simulink model "tesst"  (R2017b)
settings: Solver=FixedStepAuto  StartTime=0.0  StopTime=20  FixedStep=0.01  RelTol=1e-3
settings Model: Creator=DELL  LastModifiedBy=DELL

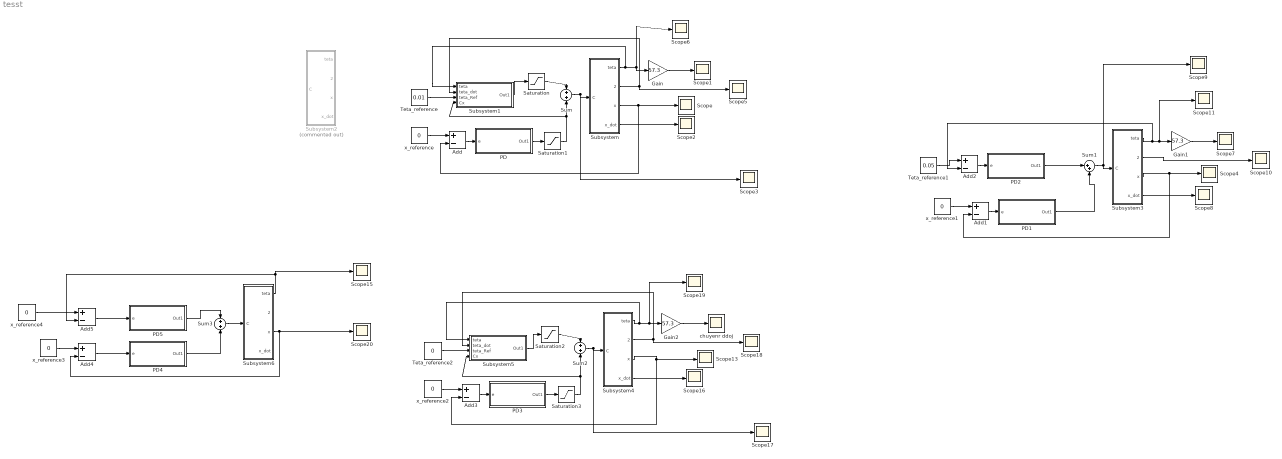
== system tesst ==
  Add{,1..5} (6 alike) : Sum  Inputs=+-
  Gain : Gain  Gain=57.3
  Gain1 : Gain  Gain=57.3
  Gain2 : Gain  Gain=57.3
  PD : Subsystem
  PD1 : Subsystem
  PD2 : Subsystem
  PD3 : Subsystem
  PD4 : Subsystem
  PD5 : Subsystem
  Saturation : Saturate  UpperLimit=0.8  LowerLimit=-0.8
  Saturation1 : Saturate  UpperLimit=0.2  LowerLimit=-0.2
  Saturation2 : Saturate  UpperLimit=0.7  LowerLimit=-0.7
  Saturation3 : Saturate  UpperLimit=0.25  LowerLimit=-0.25
  Scope{,1..11,13,15..20} (19 alike) : Scope
  Subsystem : Subsystem
  Subsystem1 : Subsystem
  Subsystem2 : Subsystem  Commented=on
  Subsystem3 : Subsystem
  Subsystem4 : Subsystem
  Subsystem5 : Subsystem
  Subsystem6 : Subsystem
  Sum : Sum
  Sum1 : Sum  Inputs=|++
  Sum2 : Sum
  Sum3 : Sum
  Teta_reference : Constant  Value=0.01
  Teta_reference1 : Constant  Value=0.05
  Teta_reference2 : Constant  Value=0
  chuyenr ddoj : Scope
  x_reference{,1..4} (5 alike) : Constant  Value=0
  wires:
  Subsystem/1(teta) -> Scope6/1, Gain/1, Subsystem1/1(teta)
  Subsystem/2(teta_dot) -> Subsystem1/2(teta_dot), Scope5/1
  Teta_reference/1 -> Subsystem1/3(teta_Ref)
  Subsystem/3(x) -> Add/2, Scope/1
  Subsystem/4(x_dot) -> Scope2/1
  Gain/1 -> Scope1/1
  x_reference/1 -> Add/1
  Add/1 -> PD/1(e)
  Sum/1 -> Scope3/1, Subsystem/1(C)
  Subsystem3/4(x_dot) -> Scope8/1
  Subsystem3/2(teta_dot) -> Scope10/1
  Gain1/1 -> Scope7/1
  Subsystem3/1(teta) -> Add2/2, Scope11/1, Gain1/1
  Subsystem3/3(x) -> Add1/2, Scope4/1
  Add1/1 -> PD1/1(e)
  Sum1/1 -> Scope9/1, Subsystem3/1(C)
  x_reference1/1 -> Add1/1
  PD1/1(Out1) -> Sum1/2
  PD2/1(Out1) -> Sum1/1
  Add2/1 -> PD2/1(e)
  Teta_reference1/1 -> Add2/1
  Subsystem1/1(Out1) -> Saturation/1
  Saturation/1 -> Sum/1
  PD/1(Out1) -> Saturation1/1
  Saturation1/1 -> Subsystem1/4(Cx), Sum/2
  Teta_reference2/1 -> Subsystem5/3(teta_Ref)
  Subsystem4/4(x_dot) -> Scope16/1
  Subsystem5/1(Out1) -> Saturation2/1
  Saturation2/1 -> Sum2/1
  Subsystem4/2(teta_dot) -> Subsystem5/2(teta_dot), Scope18/1
  Gain2/1 -> chuyenr ddoj/1
  Subsystem4/3(x) -> Add3/2, Scope13/1
  Subsystem4/1(teta) -> Scope19/1, Gain2/1, Subsystem5/1(teta)
  PD3/1(Out1) -> Saturation3/1
  Saturation3/1 -> Subsystem5/4(Cx), Sum2/2
  Add3/1 -> PD3/1(e)
  x_reference2/1 -> Add3/1
  Sum2/1 -> Scope17/1, Subsystem4/1(C)
  Add4/1 -> PD4/1(e)
  x_reference3/1 -> Add4/1
  Sum3/1 -> Subsystem6/1(C)
  PD4/1(Out1) -> Sum3/2
  Subsystem6/3(x) -> Scope20/1, Add4/2
  PD5/1(Out1) -> Sum3/1
  Add5/1 -> PD5/1(e)
  x_reference4/1 -> Add5/1
  Subsystem6/1(teta) -> Add5/2, Scope15/1

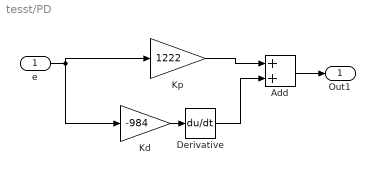
== system tesst/PD ==
  e : Inport
  Add : Sum
  Derivative : Derivative
  Kd : Gain  Gain=-984
  Kp : Gain  Gain=1222
  Out1 : Outport
  wires:
  Kp/1 -> Add/1
  e/1 -> Kd/1, Kp/1
  Add/1 -> Out1/1
  Kd/1 -> Derivative/1
  Derivative/1 -> Add/2

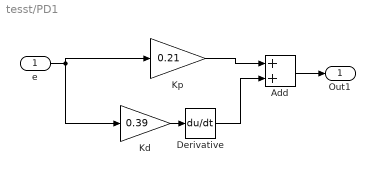
== system tesst/PD1 ==
  e : Inport
  Add : Sum
  Derivative : Derivative
  Kd : Gain  Gain=0.39
  Kp : Gain  Gain=0.21
  Out1 : Outport
  wires:
  Kp/1 -> Add/1
  e/1 -> Kd/1, Kp/1
  Add/1 -> Out1/1
  Kd/1 -> Derivative/1
  Derivative/1 -> Add/2

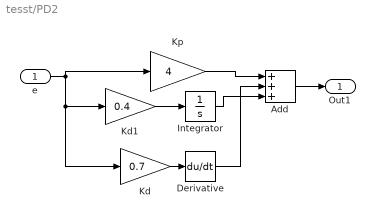
== system tesst/PD2 ==
  e : Inport
  Add : Sum  Inputs=+++
  Derivative : Derivative
  Integrator : Integrator
  Kd : Gain  Gain=0.7
  Kd1 : Gain  Gain=0.4
  Kp : Gain  Gain=4
  Out1 : Outport
  wires:
  Derivative/1 -> Add/2
  Kd/1 -> Derivative/1
  Add/1 -> Out1/1
  e/1 -> Kp/1, Kd1/1, Kd/1
  Kp/1 -> Add/1
  Kd1/1 -> Integrator/1
  Integrator/1 -> Add/3

== system tesst/PD3 ==
  e : Inport
  Add : Sum
  Derivative : Derivative
  Kd : Gain  Gain=0.39
  Kp : Gain  Gain=0.21
  Out1 : Outport
  wires:
  Kp/1 -> Add/1
  e/1 -> Kd/1, Kp/1
  Add/1 -> Out1/1
  Kd/1 -> Derivative/1
  Derivative/1 -> Add/2

== system tesst/PD4 ==
  e : Inport
  Add : Sum
  Derivative : Derivative
  Kd : Gain  Gain=0
  Kp : Gain  Gain=0
  Out1 : Outport
  wires:
  Kp/1 -> Add/1
  e/1 -> Kd/1, Kp/1
  Add/1 -> Out1/1
  Kd/1 -> Derivative/1
  Derivative/1 -> Add/2

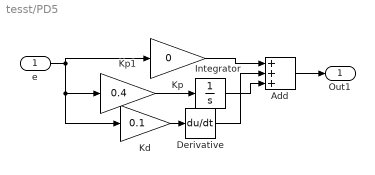
== system tesst/PD5 ==
  e : Inport
  Add : Sum  Inputs=+++
  Derivative : Derivative
  Integrator : Integrator
  Kd : Gain  Gain=0.1
  Kp : Gain  Gain=0
  Kp1 : Gain  Gain=0.4
  Out1 : Outport
  wires:
  Derivative/1 -> Add/2
  Kd/1 -> Derivative/1
  Add/1 -> Out1/1
  e/1 -> Kp/1, Kp1/1, Kd/1
  Kp/1 -> Add/1
  Kp1/1 -> Integrator/1
  Integrator/1 -> Add/3

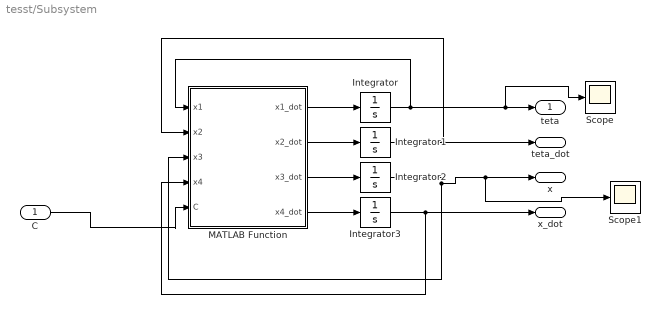
== system tesst/Subsystem ==
  C : Inport
  Integrator{,1..3} (4 alike) : Integrator
  MATLAB Function : MATLAB Function  TreatAsAtomicUnit=on
  Scope : Scope
  Scope1 : Scope
  teta : Outport
  teta_dot : Outport  Port=2
  x : Outport  Port=3
  x_dot : Outport  Port=4
  wires:
  MATLAB Function/2(x2_dot) -> Integrator1/1
  Integrator/1 -> teta/1, Scope/1, MATLAB Function/1(x1)
  MATLAB Function/4(x4_dot) -> Integrator3/1
  MATLAB Function/3(x3_dot) -> Integrator2/1
  MATLAB Function/1(x1_dot) -> Integrator/1
  Integrator1/1 -> teta_dot/1, MATLAB Function/2(x2)
  Integrator2/1 -> x/1, Scope1/1, MATLAB Function/3(x3)
  Integrator3/1 -> x_dot/1, MATLAB Function/4(x4)
  C/1 -> MATLAB Function/5(C)

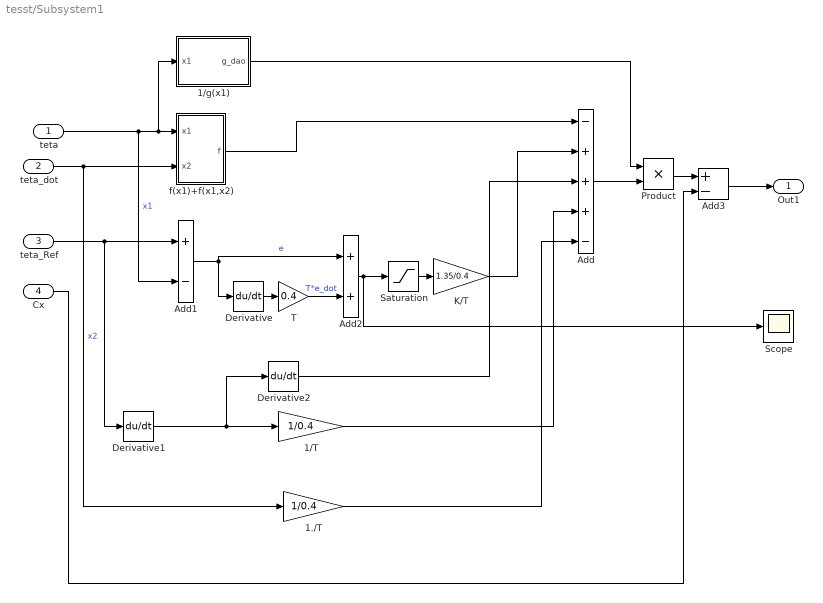
== system tesst/Subsystem1 ==
  teta : Inport
  teta_dot : Inport  Port=2
  teta_Ref : Inport  Port=3
  Cx : Inport  Port=4
  1./T : Gain  Gain=1/0.4
  1/T : Gain  Gain=1/0.4
  1/g(x1) : MATLAB Function  TreatAsAtomicUnit=on
  Add : Sum  Inputs=-+++-
  Add1 : Sum  Inputs=+-
  Add2 : Sum
  Add3 : Sum  Inputs=+-
  Derivative : Derivative
  Derivative1 : Derivative
  Derivative2 : Derivative
  K/T : Gain  Gain=1.35/0.4
  Product : Product
  Saturation : Saturate  UpperLimit=0.4  LowerLimit=-0.4
  Scope : Scope
  T : Gain  Gain=0.4
  f(x1)+f(x1,x2) : MATLAB Function  TreatAsAtomicUnit=on
  Out1 : Outport
  wires:
  teta_dot/1 -> 1./T/1, f(x1)+f(x1,x2)/2(x2)  "x2"
  teta/1 -> Add1/2, 1/g(x1)/1(x1), f(x1)+f(x1,x2)/1(x1)  "x1"
  1/g(x1)/1(g_dao) -> Product/1
  Add/1 -> Product/2
  f(x1)+f(x1,x2)/1(f) -> Add/1
  teta_Ref/1 -> Derivative1/1, Add1/1
  Derivative/1 -> T/1
  Add1/1 -> Derivative/1, Add2/1  "e"
  T/1 -> Add2/2  "T*e_dot"
  Add2/1 -> Scope/1, Saturation/1
  Saturation/1 -> K/T/1
  K/T/1 -> Add/2
  Derivative1/1 -> Derivative2/1, 1/T/1
  Derivative2/1 -> Add/3
  1/T/1 -> Add/4
  1./T/1 -> Add/5
  Product/1 -> Add3/1
  Cx/1 -> Add3/2
  Add3/1 -> Out1/1

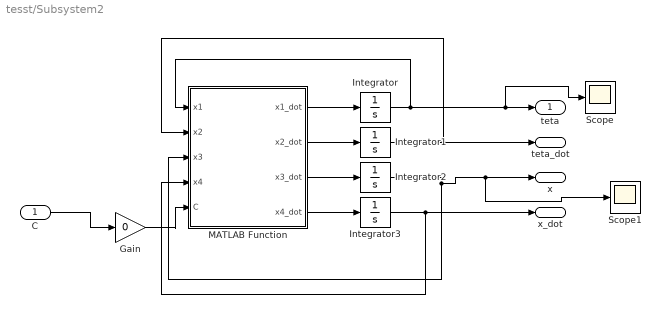
== system tesst/Subsystem2 ==
  C : Inport
  Gain : Gain  Gain=0
  Integrator : Integrator  InitialCondition=0.014
  Integrator1 : Integrator
  Integrator2 : Integrator  InitialCondition=0.03
  Integrator3 : Integrator
  MATLAB Function : MATLAB Function  TreatAsAtomicUnit=on
  Scope : Scope
  Scope1 : Scope
  teta : Outport
  teta_dot : Outport  Port=2
  x : Outport  Port=3
  x_dot : Outport  Port=4
  wires:
  MATLAB Function/2(x2_dot) -> Integrator1/1
  C/1 -> Gain/1
  Integrator/1 -> teta/1, Scope/1, MATLAB Function/1(x1)
  MATLAB Function/4(x4_dot) -> Integrator3/1
  MATLAB Function/3(x3_dot) -> Integrator2/1
  MATLAB Function/1(x1_dot) -> Integrator/1
  Integrator1/1 -> teta_dot/1, MATLAB Function/2(x2)
  Integrator2/1 -> x/1, Scope1/1, MATLAB Function/3(x3)
  Integrator3/1 -> x_dot/1, MATLAB Function/4(x4)
  Gain/1 -> MATLAB Function/5(C)

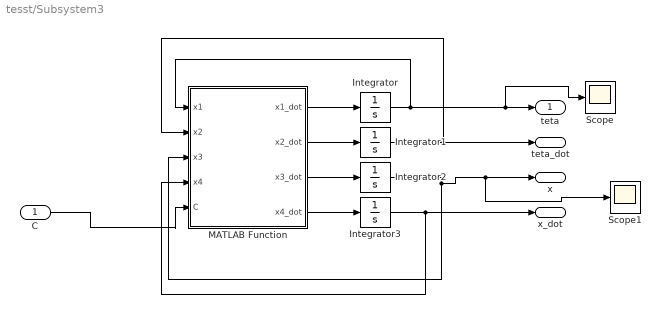
== system tesst/Subsystem3 ==
  C : Inport
  Integrator : Integrator  InitialCondition=0.014
  Integrator1 : Integrator
  Integrator2 : Integrator  InitialCondition=0.03
  Integrator3 : Integrator
  MATLAB Function : MATLAB Function  TreatAsAtomicUnit=on
  Scope : Scope
  Scope1 : Scope
  teta : Outport
  teta_dot : Outport  Port=2
  x : Outport  Port=3
  x_dot : Outport  Port=4
  wires:
  MATLAB Function/2(x2_dot) -> Integrator1/1
  Integrator/1 -> teta/1, Scope/1, MATLAB Function/1(x1)
  MATLAB Function/4(x4_dot) -> Integrator3/1
  MATLAB Function/3(x3_dot) -> Integrator2/1
  MATLAB Function/1(x1_dot) -> Integrator/1
  Integrator1/1 -> teta_dot/1, MATLAB Function/2(x2)
  Integrator2/1 -> x/1, Scope1/1, MATLAB Function/3(x3)
  Integrator3/1 -> x_dot/1, MATLAB Function/4(x4)
  C/1 -> MATLAB Function/5(C)

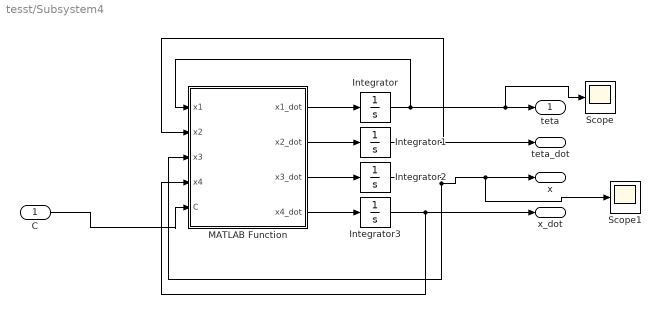
== system tesst/Subsystem4 ==
  C : Inport
  Integrator : Integrator  InitialCondition=0.017
  Integrator1 : Integrator
  Integrator2 : Integrator
  Integrator3 : Integrator
  MATLAB Function : MATLAB Function  TreatAsAtomicUnit=on
  Scope : Scope
  Scope1 : Scope
  teta : Outport
  teta_dot : Outport  Port=2
  x : Outport  Port=3
  x_dot : Outport  Port=4
  wires:
  MATLAB Function/2(x2_dot) -> Integrator1/1
  Integrator/1 -> teta/1, Scope/1, MATLAB Function/1(x1)
  MATLAB Function/4(x4_dot) -> Integrator3/1
  MATLAB Function/3(x3_dot) -> Integrator2/1
  MATLAB Function/1(x1_dot) -> Integrator/1
  Integrator1/1 -> teta_dot/1, MATLAB Function/2(x2)
  Integrator2/1 -> x/1, Scope1/1, MATLAB Function/3(x3)
  Integrator3/1 -> x_dot/1, MATLAB Function/4(x4)
  C/1 -> MATLAB Function/5(C)

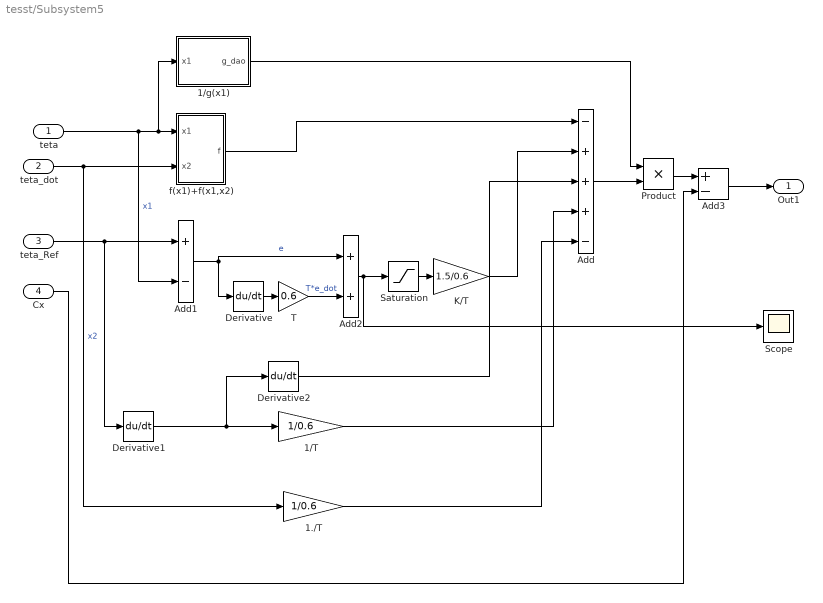
== system tesst/Subsystem5 ==
  teta : Inport
  teta_dot : Inport  Port=2
  teta_Ref : Inport  Port=3
  Cx : Inport  Port=4
  1./T : Gain  Gain=1/0.6
  1/T : Gain  Gain=1/0.6
  1/g(x1) : MATLAB Function  TreatAsAtomicUnit=on
  Add : Sum  Inputs=-+++-
  Add1 : Sum  Inputs=+-
  Add2 : Sum
  Add3 : Sum  Inputs=+-
  Derivative : Derivative
  Derivative1 : Derivative
  Derivative2 : Derivative
  K/T : Gain  Gain=1.5/0.6
  Product : Product
  Saturation : Saturate  UpperLimit=0.4  LowerLimit=-0.4
  Scope : Scope
  T : Gain  Gain=0.6
  f(x1)+f(x1,x2) : MATLAB Function  TreatAsAtomicUnit=on
  Out1 : Outport
  wires:
  teta_dot/1 -> 1./T/1, f(x1)+f(x1,x2)/2(x2)  "x2"
  teta/1 -> Add1/2, 1/g(x1)/1(x1), f(x1)+f(x1,x2)/1(x1)  "x1"
  1/g(x1)/1(g_dao) -> Product/1
  Add/1 -> Product/2
  f(x1)+f(x1,x2)/1(f) -> Add/1
  teta_Ref/1 -> Derivative1/1, Add1/1
  Derivative/1 -> T/1
  Add1/1 -> Derivative/1, Add2/1  "e"
  T/1 -> Add2/2  "T*e_dot"
  Add2/1 -> Scope/1, Saturation/1
  Saturation/1 -> K/T/1
  K/T/1 -> Add/2
  Derivative1/1 -> Derivative2/1, 1/T/1
  Derivative2/1 -> Add/3
  1/T/1 -> Add/4
  1./T/1 -> Add/5
  Product/1 -> Add3/1
  Cx/1 -> Add3/2
  Add3/1 -> Out1/1

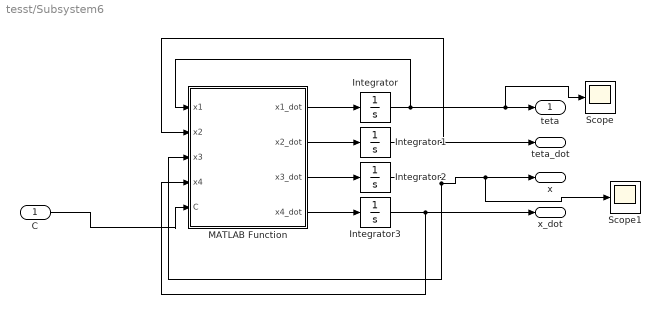
== system tesst/Subsystem6 ==
  C : Inport
  Integrator : Integrator  InitialCondition=0.017
  Integrator1 : Integrator
  Integrator2 : Integrator
  Integrator3 : Integrator
  MATLAB Function : MATLAB Function  TreatAsAtomicUnit=on
  Scope : Scope
  Scope1 : Scope
  teta : Outport
  teta_dot : Outport  Port=2
  x : Outport  Port=3
  x_dot : Outport  Port=4
  wires:
  MATLAB Function/2(x2_dot) -> Integrator1/1
  Integrator/1 -> teta/1, Scope/1, MATLAB Function/1(x1)
  MATLAB Function/4(x4_dot) -> Integrator3/1
  MATLAB Function/3(x3_dot) -> Integrator2/1
  MATLAB Function/1(x1_dot) -> Integrator/1
  Integrator1/1 -> teta_dot/1, MATLAB Function/2(x2)
  Integrator2/1 -> x/1, Scope1/1, MATLAB Function/3(x3)
  Integrator3/1 -> x_dot/1, MATLAB Function/4(x4)
  C/1 -> MATLAB Function/5(C)

== matlab function tesst/Subsystem1/f(x1)+f(x1,x2) ==
  data: x1 input; f output; x2 input
function f = fcn(x1,x2)
Mw=0.5;
Mb=7;
R=0.07;
L=0.3;
D=0.41;
g=9.8;
f=(-0.75*g*sin(x1)/L)/((0.75*(Mw*R+Mb*L*cos(x1))*cos(x1)/((2*Mw+Mb)*L))-1)+...
    (0.75*Mb*L*sin(x1)*cos(x1)*(x2^2)/(L*(2*Mw+Mb)))/((0.75*(Mw*R+Mb*L*cos(x1))*cos(x1)/((2*Mw+Mb)*L))-1);

== matlab function tesst/Subsystem/MATLAB Function ==
  data: x1 input; x1_dot output; x2 input; x3 input; x4 input; C input; x2_dot output; x3_dot output; x4_dot output
function [x1_dot,x2_dot,x3_dot,x4_dot] = fcn(x1,x2,x3,x4,C)
Mw=0.5;
Mb=7;
R=0.07;
L=0.3;
D=0.41;
g=9.8;
x1_dot=x2;
x2_dot=(-0.75*g*sin(x1)/L)/((0.75*(Mw*R+Mb*L*cos(x1))*cos(x1)/((2*Mw+Mb)*L))-1)+...
    (0.75*Mb*L*sin(x1)*cos(x1)*(x2^2)/(L*(2*Mw+Mb)))/((0.75*(Mw*R+Mb*L*cos(x1))*cos(x1)/((2*Mw+Mb)*L))-1)+...
 C*(0.75*(Mw*R+Mb*L*cos(x1))*(1+(sin(x1)^2))/(Mb*L^2)+1/R)/(2*Mw+Mb-(0.75*(Mw*R+Mb*L*cos(x1))*cos(x1)/L));


x3_dot=x4;
x4_dot=(-0.75*g*(Mw*R+Mb*L*cos(x1))*sin(x1)/L)/(2*Mw+Mb-(0.75*(Mw*R+Mb*L*cos(x1))*cos(x1)/L))+...
    (Mb*L*sin(x1)*(x2^2))/((2*Mw+Mb-(0.75*(Mw*R+Mb*L*cos(x1))*cos(x1)/L)))+...
    C*((0.75*(Mw*R+Mb*L*cos(x1))*(1+(sin(x1)^2))/(Mb*L))+(1/R))/((2*Mw+Mb-(0.75*(Mw*R+Mb*L*cos(x1))*cos(x1)/L)));

== matlab function tesst/Subsystem1/1//g(x1) ==
  data: x1 input; g_dao output
function g_dao = fcn(x1)
Mw=0.5;
Mb=7;
R=0.07;
L=0.3;
D=0.41;
g=9.8;
g_dao=1/((0.75*(Mw*R+Mb*L*cos(x1))*(1+(sin(x1)^2))/(Mb*L^2)+1/R)/(2*Mw+Mb-(0.75*(Mw*R+Mb*L*cos(x1))*cos(x1)/L)));

== matlab function tesst/Subsystem2/MATLAB Function ==
  data: x1 input; x1_dot output; x2 input; x3 input; x4 input; C input; x2_dot output; x3_dot output; x4_dot output
function [x1_dot,x2_dot,x3_dot,x4_dot] = fcn(x1,x2,x3,x4,C)
Mw=0.5;
Mb=7;
R=0.07;
L=0.3;
D=0.41;
g=9.8;
x1_dot=x2;
x2_dot=(-0.75*g*sin(x1)/L)/((0.75*(Mw*R+Mb*L*cos(x1))*cos(x1)/((2*Mw+Mb)*L))-1)+...
    (0.75*Mb*L*sin(x1)*cos(x1)*(x2^2)/(L*(2*Mw+Mb)))/((0.75*(Mw*R+Mb*L*cos(x1))*cos(x1)/((2*Mw+Mb)*L))-1)+...
 C*(0.75*(Mw*R+Mb*L*cos(x1))*(1+(sin(x1)^2))/(Mb*L^2)+1/R)/(2*Mw+Mb-(0.75*(Mw*R+Mb*L*cos(x1))*cos(x1)/L));


x3_dot=x4;
x4_dot=(-0.75*g*(Mw*R+Mb*L*cos(x1))*sin(x1)/L)/(2*Mw+Mb-(0.75*(Mw*R+Mb*L*cos(x1))*cos(x1)/L))+...
    (Mb*L*sin(x1)*(x2^2))/((2*Mw+Mb-(0.75*(Mw*R+Mb*L*cos(x1))*cos(x1)/L)))+...
    C*((0.75*(Mw*R+Mb*L*cos(x1))*(1+(sin(x1)^2))/(Mb*L))+(1/R))/((2*Mw+Mb-(0.75*(Mw*R+Mb*L*cos(x1))*cos(x1)/L)));

== matlab function tesst/Subsystem3/MATLAB Function ==
  data: x1 input; x1_dot output; x2 input; x3 input; x4 input; C input; x2_dot output; x3_dot output; x4_dot output
function [x1_dot,x2_dot,x3_dot,x4_dot] = fcn(x1,x2,x3,x4,C)
Mw=0.5;
Mb=7;
R=0.07;
L=0.3;
D=0.41;
g=9.8;
x1_dot=x2;
x2_dot=(-0.75*g*sin(x1)/L)/((0.75*(Mw*R+Mb*L*cos(x1))*cos(x1)/((2*Mw+Mb)*L))-1)+...
    (0.75*Mb*L*sin(x1)*cos(x1)*(x2^2)/(L*(2*Mw+Mb)))/((0.75*(Mw*R+Mb*L*cos(x1))*cos(x1)/((2*Mw+Mb)*L))-1)+...
 C*(0.75*(Mw*R+Mb*L*cos(x1))*(1+(sin(x1)^2))/(Mb*L^2)+1/R)/(2*Mw+Mb-(0.75*(Mw*R+Mb*L*cos(x1))*cos(x1)/L));


x3_dot=x4;
x4_dot=(-0.75*g*(Mw*R+Mb*L*cos(x1))*sin(x1)/L)/(2*Mw+Mb-(0.75*(Mw*R+Mb*L*cos(x1))*cos(x1)/L))+...
    (Mb*L*sin(x1)*(x2^2))/((2*Mw+Mb-(0.75*(Mw*R+Mb*L*cos(x1))*cos(x1)/L)))+...
    C*((0.75*(Mw*R+Mb*L*cos(x1))*(1+(sin(x1)^2))/(Mb*L))+(1/R))/((2*Mw+Mb-(0.75*(Mw*R+Mb*L*cos(x1))*cos(x1)/L)));

== matlab function tesst/Subsystem4/MATLAB Function ==
  data: x1 input; x1_dot output; x2 input; x3 input; x4 input; C input; x2_dot output; x3_dot output; x4_dot output
function [x1_dot,x2_dot,x3_dot,x4_dot] = fcn(x1,x2,x3,x4,C)
Mw=0.5;
Mb=7;
R=0.07;
L=0.3;
D=0.41;
g=9.8;
x1_dot=x2;
x2_dot=(-0.75*g*sin(x1)/L)/((0.75*(Mw*R+Mb*L*cos(x1))*cos(x1)/((2*Mw+Mb)*L))-1)+...
    (0.75*Mb*L*sin(x1)*cos(x1)*(x2^2)/(L*(2*Mw+Mb)))/((0.75*(Mw*R+Mb*L*cos(x1))*cos(x1)/((2*Mw+Mb)*L))-1)+...
 C*(0.75*(Mw*R+Mb*L*cos(x1))*(1+(sin(x1)^2))/(Mb*L^2)+1/R)/(2*Mw+Mb-(0.75*(Mw*R+Mb*L*cos(x1))*cos(x1)/L));


x3_dot=x4;
x4_dot=(-0.75*g*(Mw*R+Mb*L*cos(x1))*sin(x1)/L)/(2*Mw+Mb-(0.75*(Mw*R+Mb*L*cos(x1))*cos(x1)/L))+...
    (Mb*L*sin(x1)*(x2^2))/((2*Mw+Mb-(0.75*(Mw*R+Mb*L*cos(x1))*cos(x1)/L)))+...
    C*((0.75*(Mw*R+Mb*L*cos(x1))*(1+(sin(x1)^2))/(Mb*L))+(1/R))/((2*Mw+Mb-(0.75*(Mw*R+Mb*L*cos(x1))*cos(x1)/L)));

== matlab function tesst/Subsystem5/1//g(x1) ==
  data: x1 input; g_dao output
function g_dao = fcn(x1)
Mw=0.5;
Mb=7;
R=0.07;
L=0.3;
D=0.41;
g=9.8;
g_dao=1/((0.75*(Mw*R+Mb*L*cos(x1))*(1+(sin(x1)^2))/(Mb*L^2)+1/R)/(2*Mw+Mb-(0.75*(Mw*R+Mb*L*cos(x1))*cos(x1)/L)));

== matlab function tesst/Subsystem5/f(x1)+f(x1,x2) ==
  data: x1 input; f output; x2 input
function f = fcn(x1,x2)
Mw=0.5;
Mb=7;
R=0.07;
L=0.3;
D=0.41;
g=9.8;
f=(-0.75*g*sin(x1)/L)/((0.75*(Mw*R+Mb*L*cos(x1))*cos(x1)/((2*Mw+Mb)*L))-1)+...
    (0.75*Mb*L*sin(x1)*cos(x1)*(x2^2)/(L*(2*Mw+Mb)))/((0.75*(Mw*R+Mb*L*cos(x1))*cos(x1)/((2*Mw+Mb)*L))-1);

== matlab function tesst/Subsystem6/MATLAB Function ==
  data: x1 input; x1_dot output; x2 input; x3 input; x4 input; C input; x2_dot output; x3_dot output; x4_dot output
function [x1_dot,x2_dot,x3_dot,x4_dot] = fcn(x1,x2,x3,x4,C)
Mw=0.5;
Mb=7;
R=0.07;
L=0.3;
D=0.41;
g=9.8;
x1_dot=x2;
x2_dot=(-0.75*g*sin(x1)/L)/((0.75*(Mw*R+Mb*L*cos(x1))*cos(x1)/((2*Mw+Mb)*L))-1)+...
    (0.75*Mb*L*sin(x1)*cos(x1)*(x2^2)/(L*(2*Mw+Mb)))/((0.75*(Mw*R+Mb*L*cos(x1))*cos(x1)/((2*Mw+Mb)*L))-1)+...
 C*(0.75*(Mw*R+Mb*L*cos(x1))*(1+(sin(x1)^2))/(Mb*L^2)+1/R)/(2*Mw+Mb-(0.75*(Mw*R+Mb*L*cos(x1))*cos(x1)/L));


x3_dot=x4;
x4_dot=(-0.75*g*(Mw*R+Mb*L*cos(x1))*sin(x1)/L)/(2*Mw+Mb-(0.75*(Mw*R+Mb*L*cos(x1))*cos(x1)/L))+...
    (Mb*L*sin(x1)*(x2^2))/((2*Mw+Mb-(0.75*(Mw*R+Mb*L*cos(x1))*cos(x1)/L)))+...
    C*((0.75*(Mw*R+Mb*L*cos(x1))*(1+(sin(x1)^2))/(Mb*L))+(1/R))/((2*Mw+Mb-(0.75*(Mw*R+Mb*L*cos(x1))*cos(x1)/L)));
